simulink model "RX_SP_Blocks"  (R2020a)
settings: Solver=VariableStepAuto  StartTime=0.0  StopTime=60  RelTol=1e-3
values from neighbouring files (symbols this model uses):
  Fs = 200    [envfft.m]    (also in vmd_fftpeak.m)
undefined symbols (not defined in the file or in its folder): designMultirateFIR, ip, usb
libraries: plutoradiolib x1, dspmlti4 x1, dspfdesign x1
settings Model: Creator=prust  LastModifiedBy=Suman
settings DataIOCC: ReturnWorkspaceOutputs=off
settings DebuggingCC: ArithmeticOperatorsInVariantConditions=warning
settings SFSimCC: SimUseLocalCustomCode=off  CustomCodeUndefinedFunction=UseInterfaceOnly
settings RTWCC: RTWUseLocalCustomCode=off
settings CodeAppCC: StateflowObjectComments=on

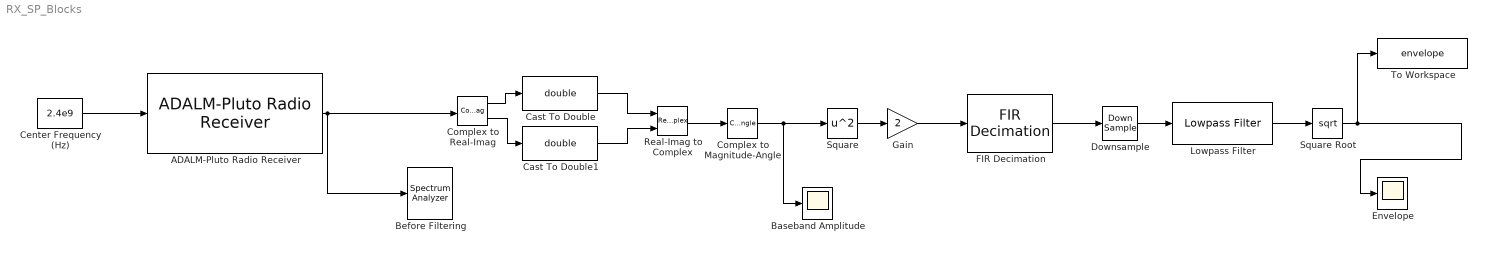
== system RX_SP_Blocks ==
  ADALM-Pluto Radio Receiver : plutoradiolib/ADALM-Pluto Radio Receiver  RadioID=usb:0  uri=ip:10.0.0.200  CenterFrequencySource=Input Port  CenterFrequency=2.4e9  GainSource=AGC Slow Attack  GainSourceBlock=Dialog  Gain=15  ChannelMapping=1  BasebandSampleRate=1e6  OutputDataType=int16  SamplesPerFrame=5000  OverflowOutputPort=off  EnableBurstMode=off  NumFramesInBurst=1  ShowAdvancedProperties=off  UseCustomFilter=off  filtPathRates=[737280000 11520000 3840000 1920000 960000 240000]  filtCoefficients=[-192 82 85 -215 228 -102 -110 290 -318 145 160 -426 471 -215 -238 633 -697 318 349 -923 1009 -457 -498 1309 -1423 640 693 -1812 1959 -876 -945 2458 -2647 1180 1268 -3290 3534 -1572 -1688 4375 -4698 2091 2247 -5836 6284 -2807 -3031 7918 -8588 3870 4225 -11182 12324 -5662 -6330 17255 -19735 9507 11312 -33568 43355 -25227 -42139 305542 305542 -42139 -25227 43355 -33568 11312 9507 -19735 17255 -6330 -5662 12324 -11182 4225 3870 -8588 7918 -3031 -2807 6284 -5836 2247 2091 -4698 4375 -1688 -1572 3534 -3290 1268 1180 -2647 2458 -945 -876 1959 -1812 693 640 -1423 1309 -498 -457 1009 -923 349 318 -697 633 -238 -215 471 -426 160 145 -318 290 -110 -102 228 -215 85 82 -192]  filtCoefficientSize=128  filtDecimInterpFactor=4  filtGain=-12  filtRFBandwidth=18000000  filterConfigStruct=struct()  EnableQuadratureCorrection=on  EnableRFDCCorrection=on  EnableBasebandDCCorrection=on  FrequencyCorrection=0  OverrideSampleTime=off  SampleTime=0.02  DataTimeout=Inf  ENSMPinControlMode=None  BISTLoopbackMode=Disabled  BISTToneInject=Disabled  BISTSignalGen=PRBS  BISTToneFreq=Fs/32  BISTToneLevel=0
      settings: SourceProductName=Communications System Toolbox Support Package for ADALM-PLUTO Radio
  Baseband Amplitude : Scope
  Before Filtering : SpectrumAnalyzer
  Cast To Double : DataTypeConversion  OutDataTypeStr=double
  Cast To Double1 : DataTypeConversion  OutDataTypeStr=double
  Center Frequency (Hz) : Constant  Value=2.4e9
  Complex to Magnitude-Angle : ComplexToMagnitudeAngle  Output=Magnitude
  Complex to Real-Imag : ComplexToRealImag
  Downsample : DownSample  N=2500
  Envelope : Scope
  FIR Decimation : dspmlti4/FIR Decimation  FilterSource=Auto  h=designMultirateFIR(1,2)  D=2  filtStruct=Direct form  FilterObject=FDECIM  InputProcessing=Columns as channels (frame based)  framing=Enforce single-rate processing  inputOffset=0  outputBufInitCond=0  roundingMode=Floor  overflowMode=off  firstCoeffDataTypeStr=Inherit: Same word length as input  firstCoeffMin=[]  firstCoeffMax=[]  firstCoeffLastDataTypeStr=Inherit: Same word length as input  outputDataTypeStr=Inherit: Same as accumulator  outputMin=[]  outputMax=[]  outputLastDataTypeStr=Inherit: Same as accumulator
  Gain : Gain  Gain=2
  Lowpass Filter : dspfdesign/Lowpass Filter  FilterType=FIR  DesignForMinimumOrder=on  FilterOrder=50  PassbandFrequency=1  StopbandFrequency=2  PassbandRipple=0.1  StopbandAttenuation=80  InheritSampleRate=off  SampleRate=200  SimulateUsing=Interpreted execution  roundingMode=Floor  coeffsDataTypeStr=fixdt(1,16)
  Real-Imag to Complex : RealImagToComplex
  Square : Math  Operator=square  OutputSignalType=real  SaturateOnIntegerOverflow=on
  Square Root : Sqrt  SaturateOnIntegerOverflow=on
  To Workspace : ToWorkspace  VariableName=envelope  SaveFormat=Timeseries  SampleTime=-1
  wires:
  Center Frequency (Hz)/1 -> ADALM-Pluto Radio Receiver/1
  Complex to Real-Imag/1 -> Cast To Double/1
  Complex to Real-Imag/2 -> Cast To Double1/1
  Cast To Double/1 -> Real-Imag to Complex/1
  Cast To Double1/1 -> Real-Imag to Complex/2
  Real-Imag to Complex/1 -> Complex to Magnitude-Angle/1
  Complex to Magnitude-Angle/1 -> Square/1, Baseband Amplitude/1
  ADALM-Pluto Radio Receiver/1 -> Complex to Real-Imag/1, Before Filtering/1
  Square/1 -> Gain/1
  Gain/1 -> FIR Decimation/1
  FIR Decimation/1 -> Downsample/1
  Downsample/1 -> Lowpass Filter/1
  Lowpass Filter/1 -> Square Root/1
  Square Root/1 -> Envelope/1, To Workspace/1
